simulink model "Predefined_time_v2"  (R2022a)
settings: Solver=ode8  StartTime=0  StopTime=1  FixedStep=1e-5  RelTol=1e-5
values from neighbouring files (symbols this model uses):
  order = 0.95    [predefined_time_M.m]
  phi_1 = (n*pi)/(4*Tc)    (= 47.1238898038)    [predefined_time_M.m]
  phi_2 = pi/(4*Tc)    (= 3.92699081699)    [predefined_time_M.m]
  phi_3 = (n*pi)/(4*Tc)    (= 47.1238898038)    [predefined_time_M.m]
  phi_4 = pi/(4*Tc)    (= 3.92699081699)    [predefined_time_M.m]
undefined symbols (not defined in the file or in its folder): phi_5, phi_6
libraries: cstblocks x32
(part 2 of 2)

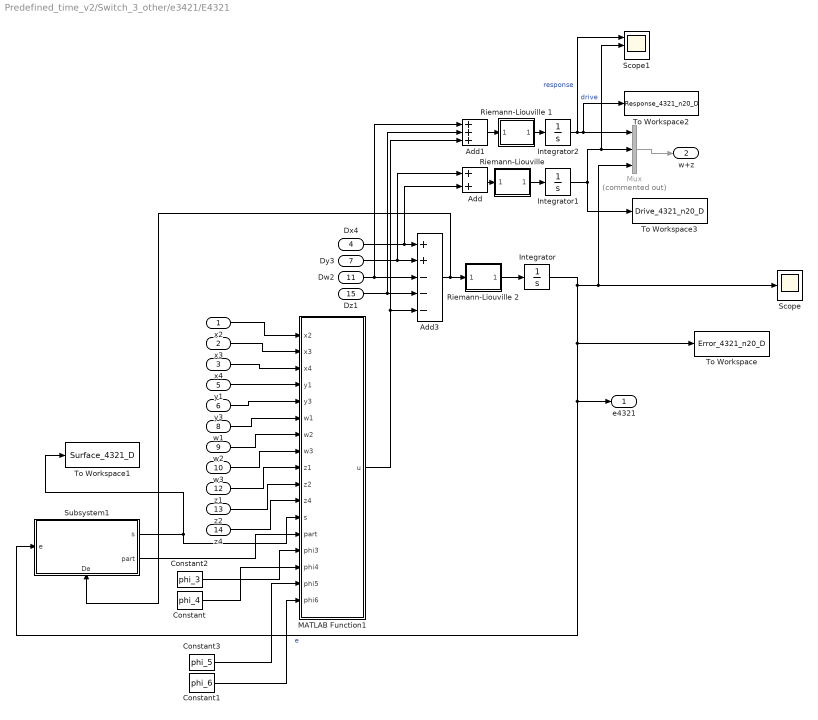
== system Predefined_time_v2/Switch_3_other/e3421/E4321 ==
  x2 : Inport
  x3 : Inport  Port=2
  x4 : Inport  Port=3
  Dx4 : Inport  Port=4
  y1 : Inport  Port=5
  y3 : Inport  Port=6
  Dy3 : Inport  Port=7
  w1 : Inport  Port=8
  w2 : Inport  Port=9
  w3 : Inport  Port=10
  Dw2 : Inport  Port=11
  z1 : Inport  Port=12
  z2 : Inport  Port=13
  z4 : Inport  Port=14
  Dz1 : Inport  Port=15
  Add : Sum
  Add1 : Sum  Inputs=+++
  Add3 : Sum  Inputs=++---
  Constant : Constant  Value=phi_4
  Constant1 : Constant  Value=phi_6
  Constant2 : Constant  Value=phi_3
  Constant3 : Constant  Value=phi_5
  Integrator : Integrator  InitialCondition=0.15
  Integrator1 : Integrator
  Integrator2 : Integrator
  MATLAB Function1 : MATLAB Function  TreatAsAtomicUnit=on
  Mux : Mux  Commented=on  Inputs=3
  "Riemann-Liouville " : Subsystem  mask{gam=1-order, ww=[1e-3, 1e3], n=5, kF1=off, kF=Oustaloup filter}
      mask prompts: gam "Derivative order gamma"; ww "Frequency range [wb,wh]"; n "Apprixmation order"; kF1 "Is a low-pass filter required?"; kF "Filter type"
      mask init: same as Predefined_time_v2/Drive system/Riemann-Liouville 1
      mask TypeOptions kF: Oustaloup filter | Modified Oustaloup filter | Matsuda-Fujii filter
      mask Display: disp(str,'texmode','on')
  Riemann-Liouville 1 : Subsystem  mask{gam=1-order, ww=[1e-3, 1e3], n=5, kF1=off, kF=Oustaloup filter}
      mask prompts: gam "Derivative order gamma"; ww "Frequency range [wb,wh]"; n "Apprixmation order"; kF1 "Is a low-pass filter required?"; kF "Filter type"
      mask init: same as Predefined_time_v2/Drive system/Riemann-Liouville 1
      mask TypeOptions kF: Oustaloup filter | Modified Oustaloup filter | Matsuda-Fujii filter
      mask Display: disp(str,'texmode','on')
  Riemann-Liouville 2 : Subsystem  mask{gam=1-order, ww=[1e-3, 1e3], n=5, kF1=off, kF=Oustaloup filter}
      mask prompts: gam "Derivative order gamma"; ww "Frequency range [wb,wh]"; n "Apprixmation order"; kF1 "Is a low-pass filter required?"; kF "Filter type"
      mask init: same as Predefined_time_v2/Drive system/Riemann-Liouville 1
      mask TypeOptions kF: Oustaloup filter | Modified Oustaloup filter | Matsuda-Fujii filter
      mask Display: disp(str,'texmode','on')
  Scope : Scope
  Scope1 : Scope  NumInputPorts=3
  Subsystem1 : Subsystem
      settings: PortSchema="{\"entries\":[{\"content\":{\"sides\":[{\"content\":{\"connectorIds\":[\"In1\"]},\"type\":\"ConnectorPlacement.EquallySpacedRectSide\",\"uuid\":\"1e5d287b-80a1-40a3-bd98-2fb678fb874f\"},{\"content\":{\"connectorIds\":[\"Out1\",\"Out2\"],\"side\":\"RIGHT\"},\"type\":\"ConnectorPlacement.EquallySpacedRectSide\",\"uuid\":\"9f557e7f-4584-4da4-ba62-067947633870\"},{\"content\":{\"connectorIds\":[],\"side\":\"TOP\"},\"type\":\"ConnectorPlacement.EquallySpacedRectSide\",\"uuid\":\"8d4dfadb-dd46-4985-a419-cdf5f3a788d3\"},{\"content\":{\"connectorIds\":[\"In2\"],\"side\":\"BOTTOM\"},\"type\":\"ConnectorPlacement.EquallySpacedRectSide\",\"uuid\":\"5511efcc-ad3c-4c5b-b8bc-b376c52e855b\"}]},\"type\":\"ConnectorPlacement.EquallySpacedConnector\",\"uuid\":\"a6ebe31d-a65f-4746-aee9-8fadd76d08af\"}],\"packageUris\":[\"http://schema.mathworks.com/mf0/Connector/R2020b\"],\"version\":\"1.0\"}"
  To Workspace : ToWorkspace  VariableName=Error_4321_n20_D  SaveFormat=Timeseries  SampleTime=-1
  To Workspace1 : ToWorkspace  VariableName=Surface_4321_D  SaveFormat=Timeseries  SampleTime=-1
  To Workspace2 : ToWorkspace  VariableName=Response_4321_n20_D  SaveFormat=Timeseries  SampleTime=-1
  To Workspace3 : ToWorkspace  VariableName=Drive_4321_n20_D  SaveFormat=Timeseries  SampleTime=-1
  e4321 : Outport
  w+z : Outport  Port=2
  wires:
  Add3/1 -> Riemann-Liouville 2/1(In1), Subsystem1/2(De)
  Dz1/1 -> Add1/2, Add3/4
  Subsystem1/1(s) -> To Workspace1/1, MATLAB Function1/12(s)
  Dw2/1 -> Add1/1, Add3/3
  Riemann-Liouville 2/1(Out1) -> Integrator/1
  Dy3/1 -> Add/1, Add3/2
  Subsystem1/2(part) -> MATLAB Function1/13(part)
  Constant/1 -> MATLAB Function1/15(phi4)
  Constant2/1 -> MATLAB Function1/14(phi3)
  Add1/1 -> Riemann-Liouville 1/1(In1)
  Riemann-Liouville 1/1(Out1) -> Integrator2/1
  Integrator2/1 -> Scope1/1, To Workspace2/1, Mux/1  "response"
  "Riemann-Liouville "/1(Out1) -> Integrator1/1
  Mux/1 -> w+z/1
  Integrator1/1 -> To Workspace3/1, Scope1/2, Mux/2  "drive"
  Add/1 -> "Riemann-Liouville "/1(In1)
  Dx4/1 -> Add/2, Add3/1
  Integrator/1 -> To Workspace/1, e4321/1, Subsystem1/1(e), Mux/3, Scope/1  "e"
  MATLAB Function1/1(u) -> Add1/3, Add3/5
  z4/1 -> MATLAB Function1/11(z4)
  z1/1 -> MATLAB Function1/9(z1)
  w2/1 -> MATLAB Function1/7(w2)
  y1/1 -> MATLAB Function1/4(y1)
  x3/1 -> MATLAB Function1/2(x3)
  x2/1 -> MATLAB Function1/1(x2)
  x4/1 -> MATLAB Function1/3(x4)
  w3/1 -> MATLAB Function1/8(w3)
  z2/1 -> MATLAB Function1/10(z2)
  w1/1 -> MATLAB Function1/6(w1)
  y3/1 -> MATLAB Function1/5(y3)
  Constant3/1 -> MATLAB Function1/16(phi5)
  Constant1/1 -> MATLAB Function1/17(phi6)

== system Predefined_time_v2/Switch_1/e3142/E3142/Riemann-Liouville  ==
  In1 : Inport
  LTI System : cstblocks/LTI System  sys=G  IC=[]
  Out1 : Outport
  wires:
  In1/1 -> LTI System/1
  LTI System/1 -> Out1/1

== system Predefined_time_v2/Switch_1/e3142/E3142/Riemann-Liouville 1 ==
  In1 : Inport
  LTI System : cstblocks/LTI System  sys=G  IC=[]
  Out1 : Outport
  wires:
  In1/1 -> LTI System/1
  LTI System/1 -> Out1/1

== system Predefined_time_v2/Switch_1/e3142/E3142/Riemann-Liouville 2 ==
  In1 : Inport
  LTI System : cstblocks/LTI System  sys=G  IC=[]
  Out1 : Outport
  wires:
  In1/1 -> LTI System/1
  LTI System/1 -> Out1/1

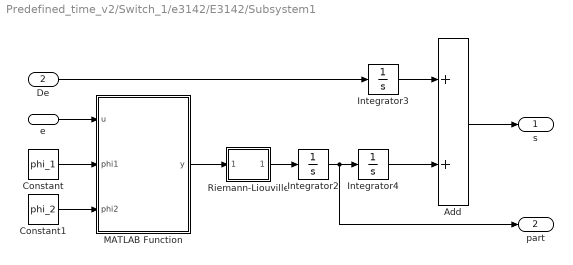
== system Predefined_time_v2/Switch_1/e3142/E3142/Subsystem1 ==
  e : Inport
  De : Inport  Port=2
  Add : Sum
  Constant : Constant  Value=phi_1
  Constant1 : Constant  Value=phi_2
  Integrator2 : Integrator
  Integrator3 : Integrator  InitialCondition=0.025
  Integrator4 : Integrator  InitialCondition=0.025
  MATLAB Function : MATLAB Function  TreatAsAtomicUnit=on
  "Riemann-Liouville " : Subsystem  mask{gam=order, ww=[1e-3, 1e3], n=5, kF1=off, kF=Oustaloup filter}
      mask prompts: gam "Derivative order gamma"; ww "Frequency range [wb,wh]"; n "Apprixmation order"; kF1 "Is a low-pass filter required?"; kF "Filter type"
      mask init: same as Predefined_time_v2/Drive system/Riemann-Liouville 1
      mask TypeOptions kF: Oustaloup filter | Modified Oustaloup filter | Matsuda-Fujii filter
      mask Display: disp(str,'texmode','on')
  s : Outport
  part : Outport  Port=2
  wires:
  Add/1 -> s/1
  Integrator3/1 -> Add/1
  "Riemann-Liouville "/1(Out1) -> Integrator2/1
  De/1 -> Integrator3/1
  MATLAB Function/1(y) -> "Riemann-Liouville "/1(In1)
  e/1 -> MATLAB Function/1(u)
  Constant1/1 -> MATLAB Function/3(phi2)
  Constant/1 -> MATLAB Function/2(phi1)
  Integrator2/1 -> part/1, Integrator4/1
  Integrator4/1 -> Add/2

== system Predefined_time_v2/Switch_2/e2314/E2314/Riemann-Liouville  ==
  In1 : Inport
  LTI System : cstblocks/LTI System  sys=G  IC=[]
  Out1 : Outport
  wires:
  In1/1 -> LTI System/1
  LTI System/1 -> Out1/1

== system Predefined_time_v2/Switch_2/e2314/E2314/Riemann-Liouville 1 ==
  In1 : Inport
  LTI System : cstblocks/LTI System  sys=G  IC=[]
  Out1 : Outport
  wires:
  In1/1 -> LTI System/1
  LTI System/1 -> Out1/1

== system Predefined_time_v2/Switch_2/e2314/E2314/Riemann-Liouville 2 ==
  In1 : Inport
  LTI System : cstblocks/LTI System  sys=G  IC=[]
  Out1 : Outport
  wires:
  In1/1 -> LTI System/1
  LTI System/1 -> Out1/1

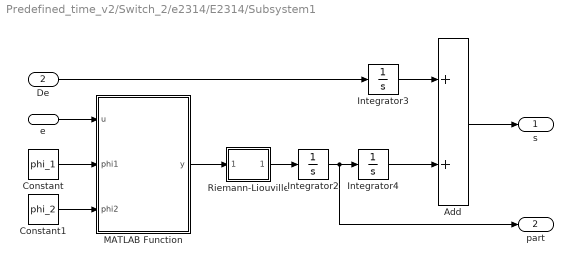
== system Predefined_time_v2/Switch_2/e2314/E2314/Subsystem1 ==
  e : Inport
  De : Inport  Port=2
  Add : Sum
  Constant : Constant  Value=phi_1
  Constant1 : Constant  Value=phi_2
  Integrator2 : Integrator
  Integrator3 : Integrator  InitialCondition=0.05
  Integrator4 : Integrator  InitialCondition=0.05
  MATLAB Function : MATLAB Function  TreatAsAtomicUnit=on
  "Riemann-Liouville " : Subsystem  mask{gam=order, ww=[1e-3, 1e3], n=5, kF1=off, kF=Oustaloup filter}
      mask prompts: gam "Derivative order gamma"; ww "Frequency range [wb,wh]"; n "Apprixmation order"; kF1 "Is a low-pass filter required?"; kF "Filter type"
      mask init: same as Predefined_time_v2/Drive system/Riemann-Liouville 1
      mask TypeOptions kF: Oustaloup filter | Modified Oustaloup filter | Matsuda-Fujii filter
      mask Display: disp(str,'texmode','on')
  s : Outport
  part : Outport  Port=2
  wires:
  Add/1 -> s/1
  Integrator3/1 -> Add/1
  "Riemann-Liouville "/1(Out1) -> Integrator2/1
  De/1 -> Integrator3/1
  MATLAB Function/1(y) -> "Riemann-Liouville "/1(In1)
  e/1 -> MATLAB Function/1(u)
  Constant1/1 -> MATLAB Function/3(phi2)
  Constant/1 -> MATLAB Function/2(phi1)
  Integrator2/1 -> part/1, Integrator4/1
  Integrator4/1 -> Add/2

== system Predefined_time_v2/Switch_3/e3421/E4321/Riemann-Liouville  ==
  In1 : Inport
  LTI System : cstblocks/LTI System  sys=G  IC=[]
  Out1 : Outport
  wires:
  In1/1 -> LTI System/1
  LTI System/1 -> Out1/1

== system Predefined_time_v2/Switch_3/e3421/E4321/Riemann-Liouville 1 ==
  In1 : Inport
  LTI System : cstblocks/LTI System  sys=G  IC=[]
  Out1 : Outport
  wires:
  In1/1 -> LTI System/1
  LTI System/1 -> Out1/1

== system Predefined_time_v2/Switch_3/e3421/E4321/Riemann-Liouville 2 ==
  In1 : Inport
  LTI System : cstblocks/LTI System  sys=G  IC=[]
  Out1 : Outport
  wires:
  In1/1 -> LTI System/1
  LTI System/1 -> Out1/1

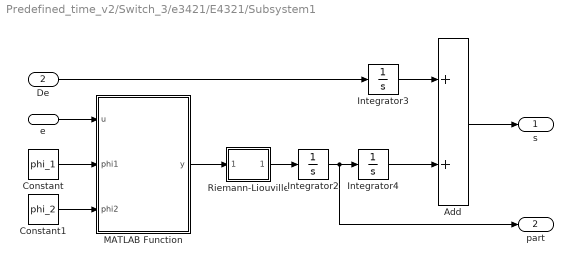
== system Predefined_time_v2/Switch_3/e3421/E4321/Subsystem1 ==
  e : Inport
  De : Inport  Port=2
  Add : Sum
  Constant : Constant  Value=phi_1
  Constant1 : Constant  Value=phi_2
  Integrator2 : Integrator
  Integrator3 : Integrator  InitialCondition=0.075
  Integrator4 : Integrator  InitialCondition=0.075
  MATLAB Function : MATLAB Function  TreatAsAtomicUnit=on
  "Riemann-Liouville " : Subsystem  mask{gam=order, ww=[1e-3, 1e3], n=5, kF1=off, kF=Oustaloup filter}
      mask prompts: gam "Derivative order gamma"; ww "Frequency range [wb,wh]"; n "Apprixmation order"; kF1 "Is a low-pass filter required?"; kF "Filter type"
      mask init: same as Predefined_time_v2/Drive system/Riemann-Liouville 1
      mask TypeOptions kF: Oustaloup filter | Modified Oustaloup filter | Matsuda-Fujii filter
      mask Display: disp(str,'texmode','on')
  s : Outport
  part : Outport  Port=2
  wires:
  Add/1 -> s/1
  Integrator3/1 -> Add/1
  "Riemann-Liouville "/1(Out1) -> Integrator2/1
  De/1 -> Integrator3/1
  MATLAB Function/1(y) -> "Riemann-Liouville "/1(In1)
  e/1 -> MATLAB Function/1(u)
  Constant1/1 -> MATLAB Function/3(phi2)
  Constant/1 -> MATLAB Function/2(phi1)
  Integrator2/1 -> part/1, Integrator4/1
  Integrator4/1 -> Add/2

== system Predefined_time_v2/Switch_3_other/e3421/E4321/Riemann-Liouville  ==
  In1 : Inport
  LTI System : cstblocks/LTI System  sys=G  IC=[]
  Out1 : Outport
  wires:
  In1/1 -> LTI System/1
  LTI System/1 -> Out1/1

== system Predefined_time_v2/Switch_3_other/e3421/E4321/Riemann-Liouville 1 ==
  In1 : Inport
  LTI System : cstblocks/LTI System  sys=G  IC=[]
  Out1 : Outport
  wires:
  In1/1 -> LTI System/1
  LTI System/1 -> Out1/1

== system Predefined_time_v2/Switch_3_other/e3421/E4321/Riemann-Liouville 2 ==
  In1 : Inport
  LTI System : cstblocks/LTI System  sys=G  IC=[]
  Out1 : Outport
  wires:
  In1/1 -> LTI System/1
  LTI System/1 -> Out1/1

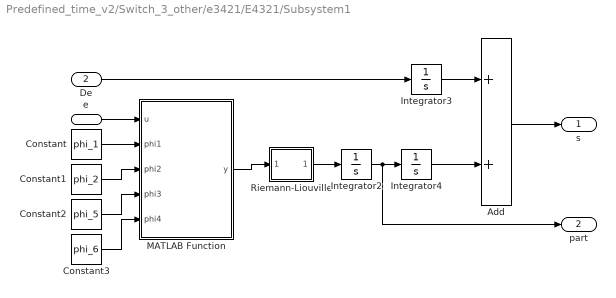
== system Predefined_time_v2/Switch_3_other/e3421/E4321/Subsystem1 ==
  e : Inport
  De : Inport  Port=2
  Add : Sum
  Constant : Constant  Value=phi_1
  Constant1 : Constant  Value=phi_2
  Constant2 : Constant  Value=phi_5
  Constant3 : Constant  Value=phi_6
  Integrator2 : Integrator
  Integrator3 : Integrator  InitialCondition=0.075
  Integrator4 : Integrator  InitialCondition=0.075
  MATLAB Function : MATLAB Function  TreatAsAtomicUnit=on
  "Riemann-Liouville " : Subsystem  mask{gam=order, ww=[1e-3, 1e3], n=5, kF1=off, kF=Oustaloup filter}
      mask prompts: gam "Derivative order gamma"; ww "Frequency range [wb,wh]"; n "Apprixmation order"; kF1 "Is a low-pass filter required?"; kF "Filter type"
      mask init: same as Predefined_time_v2/Drive system/Riemann-Liouville 1
      mask TypeOptions kF: Oustaloup filter | Modified Oustaloup filter | Matsuda-Fujii filter
      mask Display: disp(str,'texmode','on')
  s : Outport
  part : Outport  Port=2
  wires:
  Add/1 -> s/1
  Integrator3/1 -> Add/1
  "Riemann-Liouville "/1(Out1) -> Integrator2/1
  De/1 -> Integrator3/1
  MATLAB Function/1(y) -> "Riemann-Liouville "/1(In1)
  e/1 -> MATLAB Function/1(u)
  Constant1/1 -> MATLAB Function/3(phi2)
  Constant/1 -> MATLAB Function/2(phi1)
  Integrator2/1 -> part/1, Integrator4/1
  Integrator4/1 -> Add/2
  Constant2/1 -> MATLAB Function/4(phi3)
  Constant3/1 -> MATLAB Function/5(phi4)

== system Predefined_time_v2/Switch_1/e3142/E3142/Subsystem1/Riemann-Liouville  ==
  In1 : Inport
  LTI System : cstblocks/LTI System  sys=G  IC=[]
  Out1 : Outport
  wires:
  In1/1 -> LTI System/1
  LTI System/1 -> Out1/1

== system Predefined_time_v2/Switch_2/e2314/E2314/Subsystem1/Riemann-Liouville  ==
  In1 : Inport
  LTI System : cstblocks/LTI System  sys=G  IC=[]
  Out1 : Outport
  wires:
  In1/1 -> LTI System/1
  LTI System/1 -> Out1/1

== system Predefined_time_v2/Switch_3/e3421/E4321/Subsystem1/Riemann-Liouville  ==
  In1 : Inport
  LTI System : cstblocks/LTI System  sys=G  IC=[]
  Out1 : Outport
  wires:
  In1/1 -> LTI System/1
  LTI System/1 -> Out1/1

== system Predefined_time_v2/Switch_3_other/e3421/E4321/Subsystem1/Riemann-Liouville  ==
  In1 : Inport
  LTI System : cstblocks/LTI System  sys=G  IC=[]
  Out1 : Outport
  wires:
  In1/1 -> LTI System/1
  LTI System/1 -> Out1/1

== matlab function Predefined_time_v2/Switch_3/e3421/E4321/Subsystem1/MATLAB Function ==
  data: u input; y output; phi1 input; phi2 input
function y = fcn(u,phi1,phi2)

y = phi1*tanh(100*u)*exp(u*tanh(100*u))+phi2*tanh(100*u)*exp(-u*tanh(100*u));

== matlab function Predefined_time_v2/Switch_1/e3142/E3142/MATLAB Function1 ==
  data: x1 input; x2 input; x3 input; y1 input; y2 input; w2 input; w3 input; z1 input; u output; z3 input; s input; part input; phi3 input; phi4 input
function  u= fcn(x1,x2,x3,y1,y2,w2,w3,z1,z3,s,part,phi3,phi4)

u = x1*x2-3*x3-25*y1+60*y2-0.1*w2*w3-28*z1+z1*z3+...
    part + phi3*tanh(100*s)*exp(s*tanh(100*s))+phi4*tanh(100*s)*exp(-s*tanh(100*s))...
    +3;

== matlab function Predefined_time_v2/Switch_3_other/e3421/E4321/MATLAB Function1 ==
  data: x2 input; x3 input; x4 input; y1 input; y3 input; w1 input; w2 input; w3 input; z1 input; z2 input; u output; z4 input; s input; part input; phi3 input; phi4 input; phi5 input; phi6 input
function  u= fcn(x2,x3,x4,y1,y3,w1,w2,w3,z1,z2,z4,s,part,phi3,phi4,phi5,phi6)

u =x2*x3+0.3*x4+y1*y1-4*(y1+y3)+30*w2-w1*w3-10*(z2-z1)-z4+...
    part +  phi3*tanh(100*s)*(abs(s)^phi5)+phi4*tanh(100*s)*(abs(s)^phi6)...
    +3;

== matlab function Predefined_time_v2/Switch_3_other/e3421/E4321/Subsystem1/MATLAB Function ==
  data: u input; y output; phi1 input; phi2 input; phi3 input; phi4 input
function y = fcn(u,phi1,phi2,phi3,phi4)

y = phi1*tanh(100*u)*(abs(u)^phi3)+phi2*tanh(100*u)*(abs(u)^phi4);

== matlab function Predefined_time_v2/Switch_2/e2314/E2314/MATLAB Function1 ==
  data: x1 input; x2 input; x3 input; y1 input; y3 input; w1 input; w2 input; w3 input; w4 input; z1 input; u output; z3 input; z4 input; s input; part input; phi3 input; phi4 input
function  u= fcn(x1,x2,x3,y1,y3,w1,w2,w3,w4,z1,z3,z4,s,part,phi3,phi4)

u = 7*x1-x1*x3+12*x2+y1*y1-4*(y1+y3)-14*(w1-w4)+w3*w2+z1*z3-1.3*z4+...
    part + phi3*tanh(100*s)*exp(s*tanh(100*s))+phi4*tanh(100*s)*exp(-s*tanh(100*s))...
    +3;

== matlab function Predefined_time_v2/Switch_1/e3142/E3142/Subsystem1/MATLAB Function ==
  data: u input; y output; phi1 input; phi2 input
function y = fcn(u,phi1,phi2)

y = phi1*tanh(100*u)*exp(u*tanh(100*u))+phi2*tanh(100*u)*exp(-u*tanh(100*u));

== matlab function Predefined_time_v2/Switch_2/e2314/E2314/Subsystem1/MATLAB Function ==
  data: u input; y output; phi1 input; phi2 input
function y = fcn(u,phi1,phi2)

y = phi1*tanh(100*u)*exp(u*tanh(100*u))+phi2*tanh(100*u)*exp(-u*tanh(100*u));

== matlab function Predefined_time_v2/Switch_3/e3421/E4321/MATLAB Function1 ==
  data: x2 input; x3 input; x4 input; y1 input; y3 input; w1 input; w2 input; w3 input; z1 input; z2 input; u output; z4 input; s input; part input; phi3 input; phi4 input
function  u= fcn(x2,x3,x4,y1,y3,w1,w2,w3,z1,z2,z4,s,part,phi3,phi4)

u =x2*x3+0.3*x4+y1*y1-4*(y1+y3)+30*w2-w1*w3-10*(z2-z1)-z4+...
    part + phi3*tanh(100*s)*exp(s*tanh(100*s))+phi4*tanh(100*s)*exp(-(s*tanh(100*s)))...
    +3;
